simulink model "meam_simulink"  (R2020a)
settings: Solver=FixedStepAuto  StartTime=0.0  StopTime=10.0  FixedStep=0.0001  RelTol=1e-3
undefined symbols (not defined in the file): cnc_comp, ctc_switch, ctrl_at_end, ctrl_space, delta, ea_set_1, ea_set_2, ee_att_1, ee_att_2, f_des, force_ffwd, fp_1, fp_2, frc_comp, grv_comp, ip_1, ip_2, K, Kc, Kd, Kdf, Ki, Kif, Km, Kp, Kpf, orn_at_norm, prdc_frc, q_posIni, q_posIni_1, robot_model_1, robot_model_2, rpt_num_1, rpt_num_2, Sf_diag, spr_comp, switch_val, Sx_diag, tf_1, tf_2, trj_at_end, trj_profile_1, trj_profile_2, trj_space_1, trj_space_2, trj_type_1, trj_type_2
libraries: simulink x2, vrlib x1
(part 3 of 4)

== matlab function meam_simulink/Subsystem1/Comp/Friction ==
  data: robot_model input; tau_frc output size=6; qd input size=6
function tau_frc = friction(robot_model,qd)

%     tau_frc = frictionViscousModel(qd);
%     tau_frc = frictionVisCoulModel(robot_model,qd);
    tau_frc = frictionPWModel(robot_model,qd);
    
    function tau_frc = frictionPWModel(robot_model,qd)

        tau_frc = zeros(6,1);
        
        v = zeros(7,1);
        c = zeros(7,1);
        o = zeros(7,1);
        n = zeros(7,1);
        p = zeros(7,1);
        
        tau = zeros(7,1);
        vel = zeros(7,1);
        vel(1:6) = qd;
        vel(7) = qd(5)+qd(6);        

        if robot_model == 1 || robot_model == 2 || robot_model == 3
            v = [111.2  ;87.28  ;36.49  ;9.596  ;15.42  ;0.1652 ;6.564];    % Viscous
            c = [35.98  ;55.28  ;27.51  ;7.647  ;4.747  ;0.5175 ;2.805];    % Coulumb
            o = [0.9811 ;-4.794 ;-7.222 ;0.01566;0.7782 ;0.007565;-0.2884]; % Offset
%             n = [70109  ;120235 ;69500  ;15272  ;7953   ;1020   ;6193];     % Negative slop
%             p = [74033  ;101059 ;40612  ;15335  ;11066  ;1050   ;5040];     % Positive slop
%             n = [35110	;60161	;34768	;7641	;3984	;510	;3100];     % Negative slop
%             p = [37072  ;50573  ;20324  ;7672   ;5541   ;525    ;2523];     % Positive slop
%             n = [3611   ;6095   ;3510   ;773    ;412    ;51.2   ;316];     % Negative slop
%             p = [3807   ;5136   ;2065   ;776    ;568    ;52.7   ;258];     % Positive slop
            n = [461.2  ;688.0  ;383.8  ;85.91  ;55.11  ;5.265  ;37.50];     % Negative slop
            p = [480.8  ;592.1  ;239.4  ;86.22  ;70.67  ;5.416  ;31.73];     % Positive slop
        end
        
        for i = 1:7
            if (vel(i) > -1e-1 && vel(i) <= 0)
                tau(i) = n(i)*vel(i);
            elseif  (vel(i) > 0 && vel(i) <= 1e-1)
                tau(i) = p(i)*vel(i);
            else
                tau(i) = v(i)*vel(i)+c(i)*sign(vel(i))+o(i);
            end
        end
        
        tau_frc(1) = tau(1);
        tau_frc(2) = tau(2);
        tau_frc(3) = tau(3);
        tau_frc(4) = tau(4);
        tau_frc(5) = tau(5) + tau(7);
        tau_frc(6) = tau(6) + tau(7);

    end

    function tau_frc = frictionViscousModel(qd)
    
        tau_frc = zeros(6,1);
        
        if robot_model == 2 || robot_model == 3
            tau_frc(1) = 133.7*qd(1);
            tau_frc(2) = 121.8*qd(2);
            tau_frc(3) = 53.69*qd(3);
            tau_frc(4) = 14.38*qd(4);
%             tau_frc(5) = 18.39*qd(5);
%             tau_frc(6) = 14.71*qd(6);
            
            % Coupling
            tau_frc_a = 18.39*qd(5);
            tau_frc_b = 0.4887*qd(6);
            tau_frc_c = 7.44*(qd(5)+qd(6));

            tau_frc(5) = tau_frc_a + tau_frc_c;
            tau_frc(6) = tau_frc_b + tau_frc_c;
    
        end
        
    end

    % function tau_frc = frictionModel(qd)
    % 
    % 	tau_a_bl_P = [ 35, 70, 15, 6.36, 5.015867, 0.20, 0.187356 ];
    % 	tau_a_bl_N = [ -36.95, -85.95, -36.0, -6.41, -4.1, 1.18, -2.1 ];
    % 
    % 	q_dot_striebeck_P = [ 0.26, 0.078, 0.09, 0.06, 0.06, 1.10, 0.05 ];
    % 	q_dot_striebeck_N = [ 0.26, 0.3, 0.9, 0.72, 0.072, 4.0, 0.2 ];
    % 
    % 	delta_a_P = [ 0.8, 0.28, 0.35, 0.57, 0.57, 0.80, 0.30 ];
    % 	delta_a_N = [ 0.4, 0.21, 0.465, 0.5, 0.34, 1.30, 0.34 ];
    % 
    % 	c_v_P = [ 150, 132, 68, 20.737, 24.529614, 17.758244 ];
    % 	c_v_N = [ -140.0, -118.5, -58.0, -17.5, -22.0, -18.860045 ];
    % 
    % 	delta_v_P = [ 0.24, 0.352, 0.48, 0.56, 0.411378, 0.300846 ];
    % 	delta_v_N = [ 0.24, 0.28, 0.30, 0.46, 0.30, 0.315 ];
    % 
    % 	tau_v_l_P = -0.9;
    % 	tau_v_l_N = -2; %//0.08;
    % 
    % 	q_dot_l_P = 5.0;
    % 	q_dot_l_N = -8.0;
    % 
    %     tau_frc = zeros(6,1);
    %     for j = 1:4
    %         if (qd(j) > 0)
    %             tau_frc(j) = tau_a_bl_P(j)*exp(-power((qd(j)/q_dot_striebeck_P(j)), delta_a_P(j))) ...
    %                     + c_v_P(j)*power(qd(j), (1 - delta_v_P(j)));
    %         elseif (qd(j) < 0)
    %             tau_frc(j) = tau_a_bl_N(j)*exp(-power(abs(qd(j)/q_dot_striebeck_N(j)), delta_a_N(j))) ...
    %                     + c_v_N(j)*power(abs(qd(j)), (1 - delta_v_N(j)));
    %         else
    %             tau_frc(j) = 0;
    %         end
    %     end
    % 
    %     if (qd(4) > 0)
    %         tau_a = tau_a_bl_P(4)*exp(-power((qd(4)/q_dot_striebeck_P(4)), delta_a_P(4))) ...
    %                 + c_v_P(4)*power(qd(4), (1 - delta_v_P(4)));
    %     elseif (qd(4) < 0)
    %         tau_a = tau_a_bl_N(4)*exp(-power((abs(qd(4))/q_dot_striebeck_N(4)), delta_a_N(4))) ...
    %                 + c_v_N(4)*power(abs(qd(4)), (1 - delta_v_N(4)));
    %     else
    %         tau_a = 0;
    %     end
    % 
    %     if (qd(5) > 0)
    %         tau_b = tau_a_bl_P(5)*exp(-power((qd(5)/q_dot_striebeck_P(5)), delta_a_P(5))) ...
    %                 + tau_v_l_P*(1 - exp(-(qd(5)/q_dot_l_P)));
    %     elseif (qd(5) < 0)
    %         tau_b = tau_a_bl_N(5)*exp(-power((abs(qd(5))/q_dot_striebeck_N(5)), delta_a_N(5))) ...
    %                 + tau_v_l_N*(1 - exp(-abs(qd(5))/q_dot_l_N));
    %     else
    %         tau_b = 0;
    %     end
    % 
    %     qd7 = qd(4) + qd(5);
    %     if (qd7 > 0)
    %         tau_c = tau_a_bl_P(6)*exp(-power((qd7/q_dot_striebeck_P(6)), delta_a_P(6))) ...
    %                 + c_v_P(5)*power(qd7, (1 - delta_v_P(5)));
    %     elseif (qd7 < 0)
    %         tau_c = tau_a_bl_N(6)*exp(-power((abs(qd7)/q_dot_striebeck_N(6)), delta_a_N(6))) ...
    %                 + c_v_N(5)*power(abs(qd7), (1 - delta_v_N(5)));
    %     else
    %         tau_c = 0;
    %     end
    % 
    %     tau_frc(4) = tau_a + tau_c;
    %     tau_frc(5) = tau_b + tau_c;
    %     
    % end

end

== matlab function meam_simulink/Subsystem1/Comp/Gravitational ==
  data: robot_model input; ee_att input; g input; q input size=6; tau_grv output size=6
function tau_grv = grvNE(robot_model,ee_att,g,q)

    [a_i,alpha_i,d_i,thetaPlus_i] = kinematicParametersOrigin(robot_model);

    d_e = getEElength(ee_att);

    [~,Th_i] = forwardGeometry(a_i,alpha_i,d_i,thetaPlus_i+q);

    Tn_E = [1 0 0 0
            0 1 0 0
            0 0 1 d_e
            0 0 0 1];

    Th_i(:,:,end) = Th_i(:,:,end)*Tn_E;
    
    Rh_i = zeros(3,3,6+1);
    Rh_i(:,:,1:6) = Th_i(1:3,1:3,:);

    %% Inverse Dynamics
    [m_i,ri_i_ci,Ii_i] = staticInertialParameters(robot_model,ee_att);

    rh_h_i = zeros(3,1,6+1); % +1 because of prcNE
    ci_i = zeros(3,1,6);
    for i1 = 1:6
        % origin i-1 to i on frame i-1
        rh_h_i(:,:,i1) = Th_i(1:3,4,i1);
        ci_i(:,:,i1) = m_i(i1) * ri_i_ci(:,:,i1);
    end
    
    p_obj.rh_h_i = rh_h_i;
    p_obj.ri_i_ci = ri_i_ci;
    p_obj.ci_i = ci_i;
    p_obj.Ii_i = Ii_i;
    p_obj.m_i = m_i;
    q_obj.Rh_i = Rh_i;

    tau_grv = prcNE(p_obj,q_obj,zeros(6,1),zeros(6,1),g);
    
end

== matlab function meam_simulink/Robot (Stäubli RX160)/MATLAB Function ==
  data: robot_model input; ee_att input; g input; tau_i input size=6; qdd_i output size=6; q input size=6; qd input size=6
function qdd_i = drcNE(robot_model,ee_att,g,tau_i,q,qd)

    n = 6;
    
    [a_i,alpha_i,d_i,thetaPlus_i] = kinematicParametersOrigin(robot_model);

    d_e = getEElength(ee_att);

    [~,Th_i] = forwardGeometry(a_i,alpha_i,d_i,thetaPlus_i+q);

    Tn_E = [1 0 0 0
            0 1 0 0
            0 0 1 d_e
            0 0 0 1];

    Th_i(:,:,end) = Th_i(:,:,end)*Tn_E;
    
    Rh_i = zeros(3,3,n+1);
    Rh_i(:,:,1:6) = Th_i(1:3,1:3,:);

    %% Inverse Dynamics
    [m_i,ri_i_ci,Ii_i] = staticInertialParameters(robot_model,ee_att);

    rh_h_i = zeros(3,1,n+1); % +1 because of prcNE
    ci_i = zeros(3,1,n);
    for i = 1:n
        % origin i-1 to i on frame i-1
        rh_h_i(:,:,i) = Th_i(1:3,4,i);
        ci_i(:,:,i) = m_i(i) * ri_i_ci(:,:,i);
    end
    
    f_ei_i = zeros(3,1,n);
    n_ei_i = zeros(3,1,n);

    zi_i = [0;0;1];
    zzi_i = zeros(6,1,n);
    XXi_h = zeros(6,6,n);
    for i = 1:n
        zzi_i(:,:,i) = [zeros(3,1);zi_i];
        XXi_h(:,:,i) = [Rh_i(:,:,i)', -Rh_i(:,:,i)'*SkewSym(rh_h_i(:,:,i)); zeros(3,3), Rh_i(:,:,i)'];
    end

    % i) First forward recursive computations for i = 1, ..., n
    vvFbkh_h = zeros(6,1,n+1);
    gammai_i = zeros(6,1,n);
%     aaFbkh_h = zeros(6,1,n+1);
%     aaFbkh_h(:,:,1) = [-g;0;0;0];
    ff_ei_i = zeros(6,1,n);
    betah_h = zeros(6,1,n+1);
    IIh_h = zeros(6,6,n+1);
    for i = 1:n
        vvFbkh_h(:,:,i+1) = XXi_h(:,:,i)*vvFbkh_h(:,:,i) + qd(i)*zzi_i(:,:,i);
        gammai_i(:,:,i) = [Rh_i(:,:,i)'*(cross(vvFbkh_h(4:6,:,i), cross(vvFbkh_h(4:6,:,i), rh_h_i(:,:,i)))) ...
           ;cross(Rh_i(:,:,i)'*vvFbkh_h(4:6,:,i),qd(i)*zi_i)];
%         aaFbkh_h(:,:,i+1) = XXi_h(:,:,i)*aaFbkh_h(:,:,i) + qdd(i)*zzi_i(:,:,i) + gammai_i(:,:,i);
        ff_ei_i(:,:,i) = [f_ei_i(:,:,i);n_ei_i(:,:,i)];
        betah_h(:,:,i+1) = -ff_ei_i(:,:,i) ...
            - [ cross(vvFbkh_h(4:6,:,i+1), cross(vvFbkh_h(4:6,:,i+1), ci_i(:,:,i)));
                cross(vvFbkh_h(4:6,:,i+1), Ii_i(:,:,i)*vvFbkh_h(4:6,:,i+1))];
        IIh_h(:,:,i+1) = [m_i(i)*eye(3), -SkewSym(ci_i(:,:,i)); SkewSym(ci_i(:,:,i)), Ii_i(:,:,i)];
    end

    % ii) Backward recursive computations for i = n, ..., 1
    II2h_h = zeros(6,6,n+1);
    II2h_h(:,:,n+1) = IIh_h(:,:,n+1);
    beta2h_h = zeros(6,1,n+1);
    beta2h_h(:,:,n+1) = betah_h(:,:,n+1);
    H_i = zeros(n,1);
    KKi_i = zeros(6,6,n);
    alphai_i = zeros(6,1,n);
    for i = n:-1:1
        H_i(i) = zzi_i(:,:,i)'*II2h_h(:,:,i+1)*zzi_i(:,:,i);
        KKi_i(:,:,i) = II2h_h(:,:,i+1) ...
            - II2h_h(:,:,i+1)*zzi_i(:,:,i)*(1/H_i(i))*zzi_i(:,:,i)'*II2h_h(:,:,i+1);
        alphai_i(:,:,i) = KKi_i(:,:,i)*gammai_i(:,:,i) ...
            + II2h_h(:,:,i+1)*zzi_i(:,:,i)*(1/H_i(i)) ...
            *(tau_i(i)+zzi_i(:,:,i)'*beta2h_h(:,:,i+1)) - beta2h_h(:,:,i+1);
        beta2h_h(:,:,i) = betah_h(:,:,i) - XXi_h(:,:,i)'*alphai_i(:,:,i);
        II2h_h(:,:,i) = IIh_h(:,:,i) + XXi_h(:,:,i)'*KKi_i(:,:,i)*XXi_h(:,:,i);
    end

    % iii) Second forward recursive computations for i = 1, ..., n
    aai_h = zeros(6,1,n);
    qdd_i = zeros(n,1);
    aah_h = zeros(6,1,n+1);
    aah_h(:,:,1) = [-g;zeros(3,1)];
    ffi_i = zeros(6,1,n);
    for i = 1:n
        aai_h(:,:,i) = XXi_h(:,:,i)*aah_h(:,:,i);
        qdd_i(i) = (1/H_i(i))*(-zzi_i(:,:,i)'*II2h_h(:,:,i+1)*(aai_h(:,:,i) ...
            + gammai_i(:,:,i)) + tau_i(i) + zzi_i(:,:,i)'*beta2h_h(:,:,i+1));
        aah_h(:,:,i+1) = aai_h(:,:,i) + zzi_i(:,:,i)*qdd_i(i) + gammai_i(:,:,i);
    %     ffi_i(:,:,i) = KKi_i(:,:,i)*aai_h(:,:,i) + alphai_i(:,:,i);
        ffi_i(:,:,i) = II2h_h(:,:,i+1)*aah_h(:,:,i+1) - beta2h_h(:,:,i+1);
    end
    
%     p0_e = T0_h(1:3,4,n+1);
%     R0_e = T0_h(1:3,1:3,n+1);
%     XX0_e = [R0_e, SkewSym(p0_e)*R0_e; zeros(3,3), R0_e];
%     
%     aa0_e = XX0_e*aah_h(:,:,n+1);

    function S = SkewSym(r)
        S = [0, -r(3), r(2)
            r(3), 0, -r(1)
            -r(2), r(1), 0];
    end

end

== matlab function meam_simulink/Subsystem1/Comp/Jtrn ==
  data: robot_model input; ee_att input; q_pos input size=6; tau_f output size=6; f input; switch_val input; f_fbk input
function tau_f = forceTorque(robot_model,ee_att,q_pos,f,switch_val,f_fbk)

    fc_axis = 2; % task frame 1: x, 2: y, 3: z
    
    if f_fbk(fc_axis) < switch_val
        f = zeros(6,1);
    end
    
    [a_i,~,d_i,~] = kinematicParametersOrigin(robot_model);

    d_e = getEElength(ee_att);

    J_e = jacobian(a_i,d_i,d_e,q_pos);

    tau_f = J_e'*f;

% tau_f = zeros(6,1);
        
end

== matlab function meam_simulink/Subsystem1/Comp/Spring ==
  data: robot_model input; q input size=6; tau_spr output size=6
function tau_spr = spring(robot_model,q)

    % Integrated spring and friction models from feedback
    tau_spr = springModel(robot_model,q);
    
    function tau = springModel(robot_model,q)

        r = 0.08;
        L = 0.728;

        if robot_model == 2
            Pc  = 5314;
            a0  = deg2rad(-0.8458);
            k   = 23950;
        elseif robot_model == 3
            Pc  = 4897;
            a0  = deg2rad(-1.186);
            k   = 19690;
        else
            Pc  = 0;
            a0  = 0;
            k   = 0;
        end

        x0 = sqrt(r^2+(r+L)^2-2*r*(r+L)*cos(a0+q(2)))-L;

        B1E = r*sin(a0+q(2));
        A2G = ((L+r)*B1E)./(L+x0);

        % F = k*x+Pc;

        F1 = k*x0;
        F2 = Pc*ones(1,length(x0));

        tau1 = F1.*A2G;
        tau2 = F2.*A2G;

        tau = zeros(6,1);
        tau(2) = tau1 + tau2;

    end

end

== matlab function meam_simulink/Subsystem1/Dyn Trns/MATLAB Function ==
  data: robot_model input; ee_att input; u input; tau output; q input
function tau = M_hat(robot_model,ee_att,u,q)

    tau = zeros(6,1);
    
    [a_i,alpha_i,d_i,thetaPlus_i] = kinematicParametersOrigin(robot_model);

    d_e = getEElength(ee_att);

    [~,Th_i] = forwardGeometry(a_i,alpha_i,d_i,thetaPlus_i+q);

    Tn_E = [1 0 0 0
            0 1 0 0
            0 0 1 d_e
            0 0 0 1];

    Th_i(:,:,end) = Th_i(:,:,end)*Tn_E;
    
    Rh_i = zeros(3,3,6+1);
    Rh_i(:,:,1:6) = Th_i(1:3,1:3,:);

    [m_i,ri_i_ci,Ii_i] = staticInertialParameters(robot_model,ee_att);

    rh_h_i = zeros(3,1,6+1); % +1 because of prcNE
    ci_i = zeros(3,1,6);
    for j = 1:6
        % origin i-1 to i on frame i-1
        rh_h_i(:,:,j) = Th_i(1:3,4,j);
        ci_i(:,:,j) = m_i(j) * ri_i_ci(:,:,j);
    end
    
    q_obj.Rh_i = Rh_i;
    p_obj.rh_h_i = rh_h_i;
    p_obj.m_i = m_i;
    p_obj.ci_i = ci_i;
    p_obj.Ii_i = Ii_i;

    v_hat = zeros(6,1);
    M_hat = zeros(6,6);
    for j = 1:6
        if j > 1
            v_hat(j-1) = 0;
        end
        v_hat(j) = 1;
        M_hat(j,:) = prcNE(p_obj,q_obj,zeros(6,1),v_hat,zeros(3,1));
    end
    
    tau = M_hat*u;

end

== matlab function meam_simulink/Subsystem1/Error/MATLAB Function ==
  data: y output; des input; fbk input
function y = getTaskSpcError(des,fbk)

    t_posDes = des(1:3);
    t_posFbk = fbk(1:3);
    
    x_velDes = des(13:18);
    x_velFbk = fbk(13:18);
    
    e_trn = t_posDes-t_posFbk;

    r_des = [des(4:6) des(7:9) des(10:12)];
    r_fbk = [fbk(4:6) fbk(7:9) fbk(10:12)];

    e_rot = 0.5*(cross(r_fbk(:,1),r_des(:,1))+cross(r_fbk(:,2),r_des(:,2))+cross(r_fbk(:,3),r_des(:,3)));

    e_pos = [e_trn;e_rot];

    e_vel = x_velDes-x_velFbk;

    y = [e_pos;e_vel];
        
end

== matlab function meam_simulink/Subsystem1/Force Controller/D Controller ==
  data: Kd input; u input size=6; y output size=6
function y = fcn(Kd,u)

    tau = zeros(6,1);
    
    tau(1) = Kd(1)*u(1);
    tau(2) = Kd(2)*u(2);
    tau(3) = Kd(3)*u(3);
    tau(4) = Kd(4)*u(4);
    tau(5) = Kd(5)*u(5);
    tau(6) = Kd(6)*u(6);

y = tau;

== matlab function meam_simulink/Subsystem1/Force Controller/I Controller ==
  data: Ki input; u input size=6; y output size=6
function y = fcn(Ki,u)

    tau = zeros(6,1);
    
    tau(1) = Ki(1)*u(1);
    tau(2) = Ki(2)*u(2);
    tau(3) = Ki(3)*u(3);
    tau(4) = Ki(4)*u(4);
    tau(5) = Ki(5)*u(5);
    tau(6) = Ki(6)*u(6);

y = tau;

== matlab function meam_simulink/Subsystem1/Force Controller/P Controller ==
  data: Kp input; u input size=6; y output size=6
function y = fcn(Kp,u)

    tau = zeros(6,1);
    
    tau(1) = Kp(1)*u(1);
    tau(2) = Kp(2)*u(2);
    tau(3) = Kp(3)*u(3);
    tau(4) = Kp(4)*u(4);
    tau(5) = Kp(5)*u(5);
    tau(6) = Kp(6)*u(6);

y = tau;

== matlab function meam_simulink/Subsystem1/Kin Trns/MATLAB Function ==
  data: robot_model input; ee_att input; ctc_switch input; u input; tau output; q_pos input; q_vel input
function tau = kinematicTrans(robot_model,ee_att,ctc_switch,u,q_pos,q_vel)

    [a_i,~,d_i,~] = kinematicParametersOrigin(robot_model);

	d_e = getEElength(ee_att);

    if ctc_switch == 0
        J_e = jacobian(a_i,d_i,d_e,q_pos);

        tau = J_e'*u;
    else
        J_eDot = jacobianDot(a_i,d_i,d_e,q_pos,q_vel);
        J_eInv = inv_jacobian(a_i,d_i,d_e,q_pos);
        
        tau = J_eInv*(u-J_eDot*q_vel);
    end

end

== matlab function meam_simulink/Measurement1/fwd kin ==
  data: robot_model input; ee_att input; u input; y output
function y = fwdKin(robot_model,ee_att,u)

    q_pos = u(1:6);
    q_vel = u(7:12);
    
    x_pos = zeros(12,1);
    x_vel = zeros(6,1);
    
    [a_i,alpha_i,d_i,thetaPlus_i] = kinematicParametersOrigin(robot_model);
    
    d_e = getEElength(ee_att);

    [T0_h,~] = forwardGeometry(a_i,alpha_i,d_i,thetaPlus_i+q_pos);
    
    Tn_E = [1 0 0 0
            0 1 0 0
            0 0 1 d_e
            0 0 0 1];

    T0_E = T0_h(:,:,end)*Tn_E;

    t_pos = T0_E(1:3,4);

    J_e = jacobian(a_i,d_i,d_e,q_pos);
    
    r_posDC = [T0_E(1:3,1);T0_E(1:3,2);T0_E(1:3,3)];
    
    x_pos = [t_pos;r_posDC];
    x_vel = J_e*q_vel;
    
    y = [x_pos;x_vel];

end

== matlab function meam_simulink/Subsystem1/Motion Controller/D Controller ==
  data: Kd input; u input size=6; y output size=6
function y = fcn(Kd,u)

    tau = zeros(6,1);
    
    tau(1) = Kd(1)*u(1);
    tau(2) = Kd(2)*u(2);
    tau(3) = Kd(3)*u(3);
    tau(4) = Kd(4)*u(4);
    tau(5) = Kd(5)*u(5);
    tau(6) = Kd(6)*u(6);

y = tau;

== matlab function meam_simulink/Subsystem1/Motion Controller/I Controller ==
  data: Ki input; u input size=6; y output size=6
function y = fcn(Ki,u)

    tau = zeros(6,1);
    
    tau(1) = Ki(1)*u(1);
    tau(2) = Ki(2)*u(2);
    tau(3) = Ki(3)*u(3);
    tau(4) = Ki(4)*u(4);
    tau(5) = Ki(5)*u(5);
    tau(6) = Ki(6)*u(6);

y = tau;

== matlab function meam_simulink/Subsystem1/Motion Controller/P Controller ==
  data: Kp input; u input size=6; y output size=6
function y = fcn(Kp,u)

    tau = zeros(6,1);
    
    tau(1) = Kp(1)*u(1);
    tau(2) = Kp(2)*u(2);
    tau(3) = Kp(3)*u(3);
    tau(4) = Kp(4)*u(4);
    tau(5) = Kp(5)*u(5);
    tau(6) = Kp(6)*u(6);

y = tau;

== matlab function meam_simulink/Robot (Stäubli RX160L)/Friction ==
  data: robot_model input; tau_frc output size=6; qd input size=6
function tau_frc = friction(robot_model,qd)

%     tau_frc = frictionViscousModel(robot_model,qd);
%     tau_frc = frictionVisCoulModel(robot_model,qd);
    tau_frc = frictionPWModel(robot_model,qd);
    
    function tau_frc = frictionPWModel(robot_model,qd)

        tau_frc = zeros(6,1);
        
        v = zeros(7,1);
        c = zeros(7,1);
        o = zeros(7,1);
        n = zeros(7,1);
        p = zeros(7,1);
        
        tau = zeros(7,1);
        vel = zeros(7,1);
        vel(1:6) = qd;
        vel(7) = qd(5)+qd(6);        

        if robot_model == 1 || robot_model == 2 || robot_model == 3
            v = [111.2  ;87.28  ;36.49  ;9.596  ;15.42  ;0.1652 ;6.564];    % Viscous
            c = [35.98  ;55.28  ;27.51  ;7.647  ;4.747  ;0.5175 ;2.805];    % Coulumb
            o = [0.9811 ;-4.794 ;-7.222 ;0.01566;0.7782 ;0.007565;-0.2884]; % Offset
%             n = [70109  ;120235 ;69500  ;15272  ;7953   ;1020   ;6193];     % Negative slop
%             p = [74033  ;101059 ;40612  ;15335  ;11066  ;1050   ;5040];     % Positive slop
%             n = [35110	;60161	;34768	;7641	;3984	;510	;3100];     % Negative slop
%             p = [37072  ;50573  ;20324  ;7672   ;5541   ;525    ;2523];     % Positive slop
%             n = [3611   ;6095   ;3510   ;773    ;412    ;51.2   ;316];     % Negative slop
%             p = [3807   ;5136   ;2065   ;776    ;568    ;52.7   ;258];     % Positive slop
            n = [461.2  ;688.0  ;383.8  ;85.91  ;55.11  ;5.265  ;37.50];     % Negative slop
            p = [480.8  ;592.1  ;239.4  ;86.22  ;70.67  ;5.416  ;31.73];     % Positive slop
        end
        
        for i = 1:7
            if (vel(i) > -1e-1 && vel(i) <= 0)
                tau(i) = n(i)*vel(i);
            elseif  (vel(i) > 0 && vel(i) <= 1e-1)
                tau(i) = p(i)*vel(i);
            else
                tau(i) = v(i)*vel(i)+c(i)*sign(vel(i))+o(i);
            end
        end
        
        tau_frc(1) = tau(1);
        tau_frc(2) = tau(2);
        tau_frc(3) = tau(3);
        tau_frc(4) = tau(4);
        tau_frc(5) = tau(5) + tau(7);
        tau_frc(6) = tau(6) + tau(7);

    end

%     function tau_frc = frictionViscousModel(robot_model,qd)
%     
%         tau_frc = zeros(6,1);
%         
%         if robot_model == 2 || robot_model == 3
%             tau_frc(1) = 133.7*qd(1);
%             tau_frc(2) = 121.8*qd(2);
%             tau_frc(3) = 53.69*qd(3);
%             tau_frc(4) = 14.38*qd(4);
% %             tau_frc(5) = 18.39*qd(5);
% %             tau_frc(6) = 14.71*qd(6);
%             
%             % Coupling
%             tau_frc_a = 18.39*qd(5);
%             tau_frc_b = 0.4887*qd(6);
%             tau_frc_c = 7.44*(qd(5)+qd(6));
% 
%             tau_frc(5) = tau_frc_a + tau_frc_c;
%             tau_frc(6) = tau_frc_b + tau_frc_c;
%     
%         end
%         
%     end

%     function tau_frc = frictionVisCoulModel(robot_model,qd)
% 
%         tau_frc = zeros(6,1);
% 
%         if robot_model == 2
%             tau_frc(1) = 111.2*qd(1) + 35.98*sign(qd(1)) + 0.9811;
%             tau_frc(2) = 87.28*qd(2) + 55.28*sign(qd(2)) - 4.794;
%             tau_frc(3) = 36.49*qd(3) + 27.51*sign(qd(3)) - 7.222;
%             tau_frc(4) = 9.596*qd(4) + 7.647*sign(qd(4)) + 0.01566;
% 
%             % Coupling
%             tau_frc_a = 15.42*qd(5) + 4.747*sign(qd(5)) + 0.7782;
%             tau_frc_b = 0.1652*qd(6) + 0.5175*sign(qd(6)) + 0.007565;
%             tau_frc_c = 6.564*(qd(5)+qd(6)) + 2.805*sign(qd(5)+qd(6)) - 0.2884;
% 
%             tau_frc(5) = tau_frc_a + tau_frc_c;
%             tau_frc(6) = tau_frc_b + tau_frc_c;
%         end
% 
%     end

    % function tau_frc = frictionModel(qd)
    % 
    % 	tau_a_bl_P = [ 35, 70, 15, 6.36, 5.015867, 0.20, 0.187356 ];
    % 	tau_a_bl_N = [ -36.95, -85.95, -36.0, -6.41, -4.1, 1.18, -2.1 ];
    % 
    % 	q_dot_striebeck_P = [ 0.26, 0.078, 0.09, 0.06, 0.06, 1.10, 0.05 ];
    % 	q_dot_striebeck_N = [ 0.26, 0.3, 0.9, 0.72, 0.072, 4.0, 0.2 ];
    % 
    % 	delta_a_P = [ 0.8, 0.28, 0.35, 0.57, 0.57, 0.80, 0.30 ];
    % 	delta_a_N = [ 0.4, 0.21, 0.465, 0.5, 0.34, 1.30, 0.34 ];
    % 
    % 	c_v_P = [ 150, 132, 68, 20.737, 24.529614, 17.758244 ];
    % 	c_v_N = [ -140.0, -118.5, -58.0, -17.5, -22.0, -18.860045 ];
    % 
    % 	delta_v_P = [ 0.24, 0.352, 0.48, 0.56, 0.411378, 0.300846 ];
    % 	delta_v_N = [ 0.24, 0.28, 0.30, 0.46, 0.30, 0.315 ];
    % 
    % 	tau_v_l_P = -0.9;
    % 	tau_v_l_N = -2; %//0.08;
    % 
    % 	q_dot_l_P = 5.0;
    % 	q_dot_l_N = -8.0;
    % 
    %     tau_frc = zeros(6,1);
    %     for j = 1:4
    %         if (qd(j) > 0)
    %             tau_frc(j) = tau_a_bl_P(j)*exp(-power((qd(j)/q_dot_striebeck_P(j)), delta_a_P(j))) ...
    %                     + c_v_P(j)*power(qd(j), (1 - delta_v_P(j)));
    %         elseif (qd(j) < 0)
    %             tau_frc(j) = tau_a_bl_N(j)*exp(-power(abs(qd(j)/q_dot_striebeck_N(j)), delta_a_N(j))) ...
    %                     + c_v_N(j)*power(abs(qd(j)), (1 - delta_v_N(j)));
    %         else
    %             tau_frc(j) = 0;
    %         end
    %     end
    % 
    %     if (qd(4) > 0)
    %         tau_a = tau_a_bl_P(4)*exp(-power((qd(4)/q_dot_striebeck_P(4)), delta_a_P(4))) ...
    %                 + c_v_P(4)*power(qd(4), (1 - delta_v_P(4)));
    %     elseif (qd(4) < 0)
    %         tau_a = tau_a_bl_N(4)*exp(-power((abs(qd(4))/q_dot_striebeck_N(4)), delta_a_N(4))) ...
    %                 + c_v_N(4)*power(abs(qd(4)), (1 - delta_v_N(4)));
    %     else
    %         tau_a = 0;
    %     end
    % 
    %     if (qd(5) > 0)
    %         tau_b = tau_a_bl_P(5)*exp(-power((qd(5)/q_dot_striebeck_P(5)), delta_a_P(5))) ...
    %                 + tau_v_l_P*(1 - exp(-(qd(5)/q_dot_l_P)));
    %     elseif (qd(5) < 0)
    %         tau_b = tau_a_bl_N(5)*exp(-power((abs(qd(5))/q_dot_striebeck_N(5)), delta_a_N(5))) ...
    %                 + tau_v_l_N*(1 - exp(-abs(qd(5))/q_dot_l_N));
    %     else
    %         tau_b = 0;
    %     end
    % 
    %     qd7 = qd(4) + qd(5);
    %     if (qd7 > 0)
    %         tau_c = tau_a_bl_P(6)*exp(-power((qd7/q_dot_striebeck_P(6)), delta_a_P(6))) ...
    %                 + c_v_P(5)*power(qd7, (1 - delta_v_P(5)));
    %     elseif (qd7 < 0)
    %         tau_c = tau_a_bl_N(6)*exp(-power((abs(qd7)/q_dot_striebeck_N(6)), delta_a_N(6))) ...
    %                 + c_v_N(5)*power(abs(qd7), (1 - delta_v_N(5)));
    %     else
    %         tau_c = 0;
    %     end
    % 
    %     tau_frc(4) = tau_a + tau_c;
    %     tau_frc(5) = tau_b + tau_c;
    %     
    % end

end

== matlab function meam_simulink/Subsystem/Comp/Friction ==
  data: robot_model input; tau_frc output size=6; qd input size=6
function tau_frc = friction(robot_model,qd)

%     tau_frc = frictionViscousModel(qd);
%     tau_frc = frictionVisCoulModel(robot_model,qd);
    tau_frc = frictionPWModel(robot_model,qd);
    
    function tau_frc = frictionPWModel(robot_model,qd)

        tau_frc = zeros(6,1);
        
        v = zeros(7,1);
        c = zeros(7,1);
        o = zeros(7,1);
        n = zeros(7,1);
        p = zeros(7,1);
        
        tau = zeros(7,1);
        vel = zeros(7,1);
        vel(1:6) = qd;
        vel(7) = qd(5)+qd(6);        

        if robot_model == 1 || robot_model == 2 || robot_model == 3
            v = [111.2  ;87.28  ;36.49  ;9.596  ;15.42  ;0.1652 ;6.564];    % Viscous
            c = [35.98  ;55.28  ;27.51  ;7.647  ;4.747  ;0.5175 ;2.805];    % Coulumb
            o = [0.9811 ;-4.794 ;-7.222 ;0.01566;0.7782 ;0.007565;-0.2884]; % Offset
%             n = [70109  ;120235 ;69500  ;15272  ;7953   ;1020   ;6193];     % Negative slop
%             p = [74033  ;101059 ;40612  ;15335  ;11066  ;1050   ;5040];     % Positive slop
%             n = [35110	;60161	;34768	;7641	;3984	;510	;3100];     % Negative slop
%             p = [37072  ;50573  ;20324  ;7672   ;5541   ;525    ;2523];     % Positive slop
%             n = [3611   ;6095   ;3510   ;773    ;412    ;51.2   ;316];     % Negative slop
%             p = [3807   ;5136   ;2065   ;776    ;568    ;52.7   ;258];     % Positive slop
            n = [461.2  ;688.0  ;383.8  ;85.91  ;55.11  ;5.265  ;37.50];     % Negative slop
            p = [480.8  ;592.1  ;239.4  ;86.22  ;70.67  ;5.416  ;31.73];     % Positive slop
        end
        
        for i = 1:7
            if (vel(i) > -1e-1 && vel(i) <= 0)
                tau(i) = n(i)*vel(i);
            elseif  (vel(i) > 0 && vel(i) <= 1e-1)
                tau(i) = p(i)*vel(i);
            else
                tau(i) = v(i)*vel(i)+c(i)*sign(vel(i))+o(i);
            end
        end
        
        tau_frc(1) = tau(1);
        tau_frc(2) = tau(2);
        tau_frc(3) = tau(3);
        tau_frc(4) = tau(4);
        tau_frc(5) = tau(5) + tau(7);
        tau_frc(6) = tau(6) + tau(7);

    end

    function tau_frc = frictionViscousModel(qd)
    
        tau_frc = zeros(6,1);
        
        if robot_model == 2 || robot_model == 3
            tau_frc(1) = 133.7*qd(1);
            tau_frc(2) = 121.8*qd(2);
            tau_frc(3) = 53.69*qd(3);
            tau_frc(4) = 14.38*qd(4);
%             tau_frc(5) = 18.39*qd(5);
%             tau_frc(6) = 14.71*qd(6);
            
            % Coupling
            tau_frc_a = 18.39*qd(5);
            tau_frc_b = 0.4887*qd(6);
            tau_frc_c = 7.44*(qd(5)+qd(6));

            tau_frc(5) = tau_frc_a + tau_frc_c;
            tau_frc(6) = tau_frc_b + tau_frc_c;
    
        end
        
    end

    % function tau_frc = frictionModel(qd)
    % 
    % 	tau_a_bl_P = [ 35, 70, 15, 6.36, 5.015867, 0.20, 0.187356 ];
    % 	tau_a_bl_N = [ -36.95, -85.95, -36.0, -6.41, -4.1, 1.18, -2.1 ];
    % 
    % 	q_dot_striebeck_P = [ 0.26, 0.078, 0.09, 0.06, 0.06, 1.10, 0.05 ];
    % 	q_dot_striebeck_N = [ 0.26, 0.3, 0.9, 0.72, 0.072, 4.0, 0.2 ];
    % 
    % 	delta_a_P = [ 0.8, 0.28, 0.35, 0.57, 0.57, 0.80, 0.30 ];
    % 	delta_a_N = [ 0.4, 0.21, 0.465, 0.5, 0.34, 1.30, 0.34 ];
    % 
    % 	c_v_P = [ 150, 132, 68, 20.737, 24.529614, 17.758244 ];
    % 	c_v_N = [ -140.0, -118.5, -58.0, -17.5, -22.0, -18.860045 ];
    % 
    % 	delta_v_P = [ 0.24, 0.352, 0.48, 0.56, 0.411378, 0.300846 ];
    % 	delta_v_N = [ 0.24, 0.28, 0.30, 0.46, 0.30, 0.315 ];
    % 
    % 	tau_v_l_P = -0.9;
    % 	tau_v_l_N = -2; %//0.08;
    % 
    % 	q_dot_l_P = 5.0;
    % 	q_dot_l_N = -8.0;
    % 
    %     tau_frc = zeros(6,1);
    %     for j = 1:4
    %         if (qd(j) > 0)
    %             tau_frc(j) = tau_a_bl_P(j)*exp(-power((qd(j)/q_dot_striebeck_P(j)), delta_a_P(j))) ...
    %                     + c_v_P(j)*power(qd(j), (1 - delta_v_P(j)));
    %         elseif (qd(j) < 0)
    %             tau_frc(j) = tau_a_bl_N(j)*exp(-power(abs(qd(j)/q_dot_striebeck_N(j)), delta_a_N(j))) ...
    %                     + c_v_N(j)*power(abs(qd(j)), (1 - delta_v_N(j)));
    %         else
    %             tau_frc(j) = 0;
    %         end
    %     end
    % 
    %     if (qd(4) > 0)
    %         tau_a = tau_a_bl_P(4)*exp(-power((qd(4)/q_dot_striebeck_P(4)), delta_a_P(4))) ...
    %                 + c_v_P(4)*power(qd(4), (1 - delta_v_P(4)));
    %     elseif (qd(4) < 0)
    %         tau_a = tau_a_bl_N(4)*exp(-power((abs(qd(4))/q_dot_striebeck_N(4)), delta_a_N(4))) ...
    %                 + c_v_N(4)*power(abs(qd(4)), (1 - delta_v_N(4)));
    %     else
    %         tau_a = 0;
    %     end
    % 
    %     if (qd(5) > 0)
    %         tau_b = tau_a_bl_P(5)*exp(-power((qd(5)/q_dot_striebeck_P(5)), delta_a_P(5))) ...
    %                 + tau_v_l_P*(1 - exp(-(qd(5)/q_dot_l_P)));
    %     elseif (qd(5) < 0)
    %         tau_b = tau_a_bl_N(5)*exp(-power((abs(qd(5))/q_dot_striebeck_N(5)), delta_a_N(5))) ...
    %                 + tau_v_l_N*(1 - exp(-abs(qd(5))/q_dot_l_N));
    %     else
    %         tau_b = 0;
    %     end
    % 
    %     qd7 = qd(4) + qd(5);
    %     if (qd7 > 0)
    %         tau_c = tau_a_bl_P(6)*exp(-power((qd7/q_dot_striebeck_P(6)), delta_a_P(6))) ...
    %                 + c_v_P(5)*power(qd7, (1 - delta_v_P(5)));
    %     elseif (qd7 < 0)
    %         tau_c = tau_a_bl_N(6)*exp(-power((abs(qd7)/q_dot_striebeck_N(6)), delta_a_N(6))) ...
    %                 + c_v_N(5)*power(abs(qd7), (1 - delta_v_N(5)));
    %     else
    %         tau_c = 0;
    %     end
    % 
    %     tau_frc(4) = tau_a + tau_c;
    %     tau_frc(5) = tau_b + tau_c;
    %     
    % end

end

== matlab function meam_simulink/Robot (Stäubli RX160L)/Jtrn ==
  data: robot_model input; ee_att input; q_pos input size=6; tau_f output size=6; f input
function tau_f = forceTorque(robot_model,ee_att,q_pos,f)

    [a_i,~,d_i,~] = kinematicParametersOrigin(robot_model);

    d_e = getEElength(ee_att);

    J_e = jacobian(a_i,d_i,d_e,q_pos);

    tau_f = J_e'*f;

% tau_f = zeros(6,1);
        
end

== matlab function meam_simulink/Robot (Stäubli RX160L)/MATLAB Function ==
  data: robot_model input; ee_att input; g input; tau_i input size=6; qdd_i output size=6; q input size=6; qd input size=6
function qdd_i = drcNE(robot_model,ee_att,g,tau_i,q,qd)

    n = 6;
    
    [a_i,alpha_i,d_i,thetaPlus_i] = kinematicParametersOrigin(robot_model);

    d_e = getEElength(ee_att);

    [~,Th_i] = forwardGeometry(a_i,alpha_i,d_i,thetaPlus_i+q);

    Tn_E = [1 0 0 0
            0 1 0 0
            0 0 1 d_e
            0 0 0 1];

    Th_i(:,:,end) = Th_i(:,:,end)*Tn_E;
    
    Rh_i = zeros(3,3,n+1);
    Rh_i(:,:,1:6) = Th_i(1:3,1:3,:);

    %% Inverse Dynamics
    [m_i,ri_i_ci,Ii_i] = staticInertialParameters(robot_model,ee_att);

    rh_h_i = zeros(3,1,n+1); % +1 because of prcNE
    ci_i = zeros(3,1,n);
    for i = 1:n
        % origin i-1 to i on frame i-1
        rh_h_i(:,:,i) = Th_i(1:3,4,i);
        ci_i(:,:,i) = m_i(i) * ri_i_ci(:,:,i);
    end
    
    f_ei_i = zeros(3,1,n);
    n_ei_i = zeros(3,1,n);

    zi_i = [0;0;1];
    zzi_i = zeros(6,1,n);
    XXi_h = zeros(6,6,n);
    for i = 1:n
        zzi_i(:,:,i) = [zeros(3,1);zi_i];
        XXi_h(:,:,i) = [Rh_i(:,:,i)', -Rh_i(:,:,i)'*SkewSym(rh_h_i(:,:,i)); zeros(3,3), Rh_i(:,:,i)'];
    end

    % i) First forward recursive computations for i = 1, ..., n
    vvFbkh_h = zeros(6,1,n+1);
    gammai_i = zeros(6,1,n);
%     aaFbkh_h = zeros(6,1,n+1);
%     aaFbkh_h(:,:,1) = [-g;0;0;0];
    ff_ei_i = zeros(6,1,n);
    betah_h = zeros(6,1,n+1);
    IIh_h = zeros(6,6,n+1);
    for i = 1:n
        vvFbkh_h(:,:,i+1) = XXi_h(:,:,i)*vvFbkh_h(:,:,i) + qd(i)*zzi_i(:,:,i);
        gammai_i(:,:,i) = [Rh_i(:,:,i)'*(cross(vvFbkh_h(4:6,:,i), cross(vvFbkh_h(4:6,:,i), rh_h_i(:,:,i)))) ...
           ;cross(Rh_i(:,:,i)'*vvFbkh_h(4:6,:,i),qd(i)*zi_i)];
%         aaFbkh_h(:,:,i+1) = XXi_h(:,:,i)*aaFbkh_h(:,:,i) + qdd(i)*zzi_i(:,:,i) + gammai_i(:,:,i);
        ff_ei_i(:,:,i) = [f_ei_i(:,:,i);n_ei_i(:,:,i)];
        betah_h(:,:,i+1) = -ff_ei_i(:,:,i) ...
            - [ cross(vvFbkh_h(4:6,:,i+1), cross(vvFbkh_h(4:6,:,i+1), ci_i(:,:,i)));
                cross(vvFbkh_h(4:6,:,i+1), Ii_i(:,:,i)*vvFbkh_h(4:6,:,i+1))];
        IIh_h(:,:,i+1) = [m_i(i)*eye(3), -SkewSym(ci_i(:,:,i)); SkewSym(ci_i(:,:,i)), Ii_i(:,:,i)];
    end

    % ii) Backward recursive computations for i = n, ..., 1
    II2h_h = zeros(6,6,n+1);
    II2h_h(:,:,n+1) = IIh_h(:,:,n+1);
    beta2h_h = zeros(6,1,n+1);
    beta2h_h(:,:,n+1) = betah_h(:,:,n+1);
    H_i = zeros(n,1);
    KKi_i = zeros(6,6,n);
    alphai_i = zeros(6,1,n);
    for i = n:-1:1
        H_i(i) = zzi_i(:,:,i)'*II2h_h(:,:,i+1)*zzi_i(:,:,i);
        KKi_i(:,:,i) = II2h_h(:,:,i+1) ...
            - II2h_h(:,:,i+1)*zzi_i(:,:,i)*(1/H_i(i))*zzi_i(:,:,i)'*II2h_h(:,:,i+1);
        alphai_i(:,:,i) = KKi_i(:,:,i)*gammai_i(:,:,i) ...
            + II2h_h(:,:,i+1)*zzi_i(:,:,i)*(1/H_i(i)) ...
            *(tau_i(i)+zzi_i(:,:,i)'*beta2h_h(:,:,i+1)) - beta2h_h(:,:,i+1);
        beta2h_h(:,:,i) = betah_h(:,:,i) - XXi_h(:,:,i)'*alphai_i(:,:,i);
        II2h_h(:,:,i) = IIh_h(:,:,i) + XXi_h(:,:,i)'*KKi_i(:,:,i)*XXi_h(:,:,i);
    end

    % iii) Second forward recursive computations for i = 1, ..., n
    aai_h = zeros(6,1,n);
    qdd_i = zeros(n,1);
    aah_h = zeros(6,1,n+1);
    aah_h(:,:,1) = [-g;zeros(3,1)];
    ffi_i = zeros(6,1,n);
    for i = 1:n
        aai_h(:,:,i) = XXi_h(:,:,i)*aah_h(:,:,i);
        qdd_i(i) = (1/H_i(i))*(-zzi_i(:,:,i)'*II2h_h(:,:,i+1)*(aai_h(:,:,i) ...
            + gammai_i(:,:,i)) + tau_i(i) + zzi_i(:,:,i)'*beta2h_h(:,:,i+1));
        aah_h(:,:,i+1) = aai_h(:,:,i) + zzi_i(:,:,i)*qdd_i(i) + gammai_i(:,:,i);
    %     ffi_i(:,:,i) = KKi_i(:,:,i)*aai_h(:,:,i) + alphai_i(:,:,i);
        ffi_i(:,:,i) = II2h_h(:,:,i+1)*aah_h(:,:,i+1) - beta2h_h(:,:,i+1);
    end
    
%     p0_e = T0_h(1:3,4,n+1);
%     R0_e = T0_h(1:3,1:3,n+1);
%     XX0_e = [R0_e, SkewSym(p0_e)*R0_e; zeros(3,3), R0_e];
%     
%     aa0_e = XX0_e*aah_h(:,:,n+1);

    function S = SkewSym(r)
        S = [0, -r(3), r(2)
            r(3), 0, -r(1)
            -r(2), r(1), 0];
    end

end

== matlab function meam_simulink/Robot (Stäubli RX160L)/Spring ==
  data: robot_model input; q input size=6; tau_spr output size=6
function tau_spr = spring(robot_model,q)

    % Integrated spring and friction models from feedback
    tau_spr = springModel(robot_model,q);
    
    function tau = springModel(robot_model,q)

        r = 0.08;
        L = 0.728;

        if robot_model == 2
            Pc  = 5314;
            a0  = deg2rad(-0.8458);
            k   = 23950;
        elseif robot_model == 3
            Pc  = 4897;
            a0  = deg2rad(-1.186);
            k   = 19690;
        else
            Pc  = 0;
            a0  = 0;
            k   = 0;
        end

        x0 = sqrt(r^2+(r+L)^2-2*r*(r+L)*cos(a0+q(2)))-L;

        B1E = r*sin(a0+q(2));
        A2G = ((L+r)*B1E)./(L+x0);

        % F = k*x+Pc;

        F1 = k*x0;
        F2 = Pc*ones(1,length(x0));

        tau1 = F1.*A2G;
        tau2 = F2.*A2G;

        tau = zeros(6,1);
        tau(2) = tau1 + tau2;

    end

end

== matlab function meam_simulink/Robot (Stäubli RX160L)/fwd kin ==
  data: robot_model input; ee_att input; u input; y output
function y = fwdKin(robot_model,ee_att,u)

    q_pos = u(1:6);
    q_vel = u(7:12);
    
    [a_i,alpha_i,d_i,thetaPlus_i] = kinematicParametersOrigin(robot_model);
    
    d_e = getEElength(ee_att);

    [T0_h,~] = forwardGeometry(a_i,alpha_i,d_i,thetaPlus_i+q_pos);
    
    Tn_E = [1 0 0 0
            0 1 0 0
            0 0 1 d_e
            0 0 0 1];

    T0_E = T0_h(:,:,end)*Tn_E;

    t_pos = T0_E(1:3,4);

    J_e = jacobian(a_i,d_i,d_e,q_pos);
    
    r_posDC = [T0_E(1:3,1);T0_E(1:3,2);T0_E(1:3,3)];
    
    x_pos = [t_pos;r_posDC];
    x_vel = J_e*q_vel;
    
    y = [x_pos;x_vel];

%     function x = spring_model_func(f)
% 
%         p1 =   2.015e-13;
%         p2 =   7.036e-11;
%         p3 =   9.407e-09;
%         p4 =    5.66e-07;
%         p5 =   1.201e-05;
%         p6 =    0.000136;
%         p7 =  -1.792e-07;
% 
%         if f >= 0
%             x = 0;
%         elseif f >= -109.743
%             x = p1*f^6+p2*f^5+p3*f^4+p4*f^3+p5*f^2+p6*f+p7;
%         else
%             x = -0.0219;
%         end
% 
%     end
end

== matlab function meam_simulink/Animation/fwd kin1 ==
  data: u input; r1 output; r2 output; r3 output; r4 output; r5 output; r6 output
function [r1,r2,r3,r4,r5,r6] = fcn(u)

%     [a_i,~,d_i,~] = kinematicParametersOrigin(robot_model);

    r1 = [0;1; 0;u(1)];
    r2 = [0;0;-1;u(2)];
    r3 = [0;0;-1;u(3)];
    r4 = [0;1; 0;u(4)];
    r5 = [0;0;-1;u(5)];
    r6 = [0;1; 0;u(6)];

%     t1 = [0         d_i(1)  0]';
%     t2 = [a_i(2)    0       0]';
%     t3 = [0         a_i(3)	0]';
%     t4 = [0         0       0]';
%     t5 = [0         d_i(4)  0]';
%     t6 = [0         d_i(6)  0]';

end

== matlab function meam_simulink/Subsystem/End-to-Base/spatialTrnsE2B ==
  data: q input; x input; v input; y output; ctc_switch input; u input
function y = sptTrnsWrnE2B(q,x,v,ctc_switch,u)
    
    R_mat = [x(4:6) x(7:9) x(10:12)];
    X_r = [R_mat zeros(3,3);zeros(3,3) R_mat];
    
    if ctc_switch == 0        
        y = X_r*u;
    else        
        q_pos = q(1:6);
        q_vel = q(7:12);
    
        R_dot = getR0_6dotMatrix(q_pos,q_vel);
        X_r_dot = [R_dot zeros(3,3);zeros(3,3) R_dot];
    
        y = X_r*u + X_r_dot*X_r*v;
    end
    
end

== matlab function meam_simulink/Subsystem/Base-to-End/spatialTrnsB2E ==
  data: x input; y output; e input
function y = sptTrnsErrorB2E(x,e)
    
    R_mat = [x(4:6) x(7:9) x(10:12)];
    
    X_r_inv = [R_mat' zeros(3,3);zeros(3,3) R_mat'];
    
    y = [X_r_inv*e(1:6);X_r_inv*e(7:12)];
    
end

== matlab function meam_simulink/Environment/MATLAB Function1 ==
  data: x1 input; ee_att_1 input; x2 input size=18; K input; f_e output
function f_e = collisionModel(x1,ee_att_1,x2,K)

    L_srf = [0.64;0.64;0.00];
    
    T0_E_1 = eye(4);
    T0_E_1(1:3,1) = x1(4:6);
    T0_E_1(1:3,2) = x1(7:9);
    T0_E_1(1:3,3) = x1(10:12);
    T0_E_1(1:3,4) = x1(1:3);

    TI_0_1 = eye(4);
    TI_E_1 = TI_0_1*T0_E_1;
    
    TE_I_1 = eye(4);
    TE_I_1(1:3,1:3) = TI_E_1(1:3,1:3)';
    TE_I_1(1:3,4) = -TI_E_1(1:3,1:3)'*TI_E_1(1:3,4);
    
    T0_E_2 = eye(4);
    T0_E_2(1:3,1) = x2(4:6);
    T0_E_2(1:3,2) = x2(7:9);
    T0_E_2(1:3,3) = x2(10:12);
    T0_E_2(1:3,4) = x2(1:3);

    TI_0_2 = [  1,0,0,-0.28
                0,1,0, 2.43
                0,0,1, 0
                0,0,0, 1	];
            
    TI_E_2 = TI_0_2*T0_E_2;
    
    o_e1 = TI_E_1(1:3,4);
    o_e2 = TI_E_2(1:3,4);  
    z_e2 = TI_E_2(1:3,3);
    
    vert_srf_rel = [vertice_2d_gen(zeros(2,1),L_srf(1:2)),ones(4,1)]*TI_E_2'*TE_I_1';

    Mxy = [0,0];
    Axy = [vert_srf_rel(1,1),vert_srf_rel(1,2)];
    Bxy = [vert_srf_rel(2,1),vert_srf_rel(2,2)];
    Cxy = [vert_srf_rel(3,1),vert_srf_rel(3,2)];
    Dxy = [vert_srf_rel(4,1),vert_srf_rel(4,2)];

    coll_xy = pointInTriangle(Axy,Bxy,Cxy,Mxy) || pointInTriangle(Axy,Cxy,Dxy,Mxy);

    D = dot(z_e2,o_e2);

    d = (z_e2(1)*o_e1(1)+z_e2(2)*o_e1(2)+z_e2(3)*o_e1(3)-D)/sqrt(z_e2(1)^2+z_e2(2)^2+z_e2(3)^2);
    
    coll_z = d < 0;
    
    if coll_xy && coll_z
        if ee_att_1 == 3 && d < 0.0219
            K_mat = [K 0 0
                     0 K 0
                     0 0 5014];

            F = T0_E_1(1:3,1:3)*K_mat*T0_E_1(1:3,1:3)'*d*z_e2;
        else
            F = -K*abs(d)*z_e2;    
        end
    
        f_e = [F(1);F(2);F(3);0;0;0];
    else
        f_e = zeros(6,1);
    end
    
    % floor
    if (o_e1(3) < -0.6)
        f_e(3) = K*(o_e1(3)-0.6);
    end
    
    function vert = vertice_2d_gen(O,L)

        vert = [O(1)-L(1)/2 O(2)-L(2)/2 0; ...
                O(1)-L(1)/2 O(2)+L(2)/2 0; ...
                O(1)+L(1)/2 O(2)+L(2)/2 0; ...
                O(1)+L(1)/2 O(2)-L(2)/2 0];

    end

    function out = pointInTriangle(P1,P2,P3,P)

        denom = ((P2(2) - P3(2))*(P1(1) - P3(1)) + (P3(1) - P2(1))*(P1(2) - P3(2)));

        a = ((P2(2) - P3(2))*(P(1) - P3(1)) + (P3(1) - P2(1))*(P(2) - P3(2))) / denom;
        b = ((P3(2) - P1(2))*(P(1) - P3(1)) + (P1(1) - P3(1))*(P(2) - P3(2))) / denom;
        c = 1 - a - b;

        out = 0 <= a && a <= 1 && 0 <= b && b <= 1 && 0 <= c && c <= 1;

    end

end

== matlab function meam_simulink/Subsystem/Comp/Spring ==
  data: robot_model input; q input size=6; tau_spr output size=6
function tau_spr = spring(robot_model,q)

    % Integrated spring and friction models from feedback
    tau_spr = springModel(robot_model,q);
    
    function tau = springModel(robot_model,q)

        r = 0.08;
        L = 0.728;

        if robot_model == 2
            Pc  = 5314;
            a0  = deg2rad(-0.8458);
            k   = 23950;
        elseif robot_model == 3
            Pc  = 4897;
            a0  = deg2rad(-1.186);
            k   = 19690;
        else
            Pc  = 0;
            a0  = 0;
            k   = 0;
        end

        x0 = sqrt(r^2+(r+L)^2-2*r*(r+L)*cos(a0+q(2)))-L;

        B1E = r*sin(a0+q(2));
        A2G = ((L+r)*B1E)./(L+x0);

        % F = k*x+Pc;

        F1 = k*x0;
        F2 = Pc*ones(1,length(x0));

        tau1 = F1.*A2G;
        tau2 = F2.*A2G;

        tau = zeros(6,1);
        tau(2) = tau1 + tau2;

    end

end

== matlab function meam_simulink/Robot (Stäubli RX160L)/x_e ==
  data: ee_att_1 input; f_vec input; y output
function y = end_point(ee_att_1,f_vec)

    f = -f_vec(2);
    
    if ee_att_1 == 3
        if f > 0
            y = [0;0;0];
        elseif f < -109.8066
            y = [0;0;0.0219];
        else            
            y = [0;0;f/5014];
        end
    else
        y = [0;0;0];
    end    
    
end

== matlab function meam_simulink/Subsystem1/Selective Sum/MATLAB Function ==
  data: um input; y output; Sx_diag input; switch_val input; Sf_diag input; uf input; f_fbk input
function y = fcn(um,Sx_diag,switch_val,Sf_diag,uf,f_fbk)
    
    y = zeros(6,1);
    Sx_i = Sx_diag;
    Sf_i = Sf_diag;

    fc_axis = 2;
    
    if f_fbk(fc_axis) < switch_val
        Sx_i(fc_axis) = 1;
        Sf_i(fc_axis) = 0;
    end
    
%     if f_fbk(1) < switch_val
%         Sx_diag(1) = 1;
%         Sf_diag(1) = 0;
%     end
%     
%     Sx_i = Sx_diag;
%     Sf_i = Sf_diag;

    for i = 1:6
        y(i) = Sx_i(i)*um(i)+Sf_i(i)*uf(i);
    end

end
